simulink model "Lead_Acid_Battery_2021"  (R2024b)
settings: Solver=VariableStepAuto  StartTime=0.0  StopTime=100  RelTol=1e-3
settings Model: Creator=10537  LastModifiedBy=10537

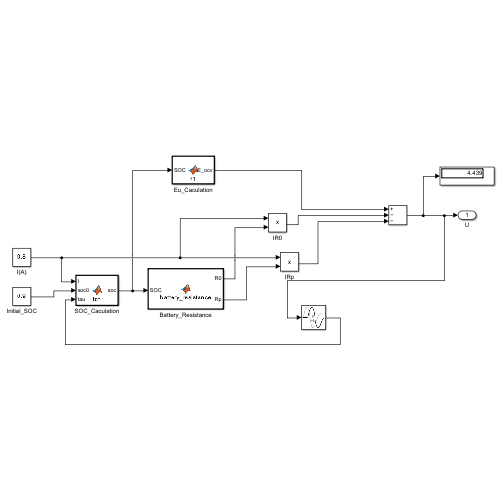
[thumbnail: Simulink's stored preview of the top-level diagram]
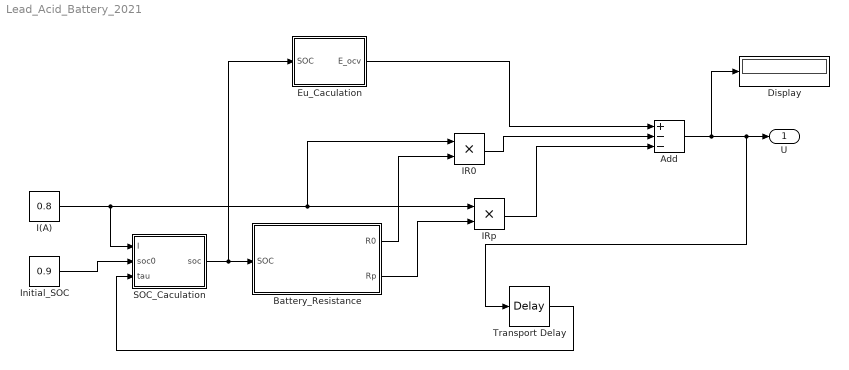
== system Lead_Acid_Battery_2021 ==
  Add : Sum  Inputs=+--
  Battery_Resistance : MATLAB Function  TreatAsAtomicUnit=on
  Display : Display
  Eu_Caculation : MATLAB Function  TreatAsAtomicUnit=on
  I(A) : Constant  Value=0.8
  IR0 : Product
  IRp : Product
  Initial_SOC : Constant  Value=0.9
  SOC_Caculation : MATLAB Function  TreatAsAtomicUnit=on
  Transport Delay : TransportDelay
  U : Outport
  wires:
  Battery_Resistance/1(R0) -> IR0/2
  Battery_Resistance/2(Rp) -> IRp/2
  IR0/1 -> Add/2
  IRp/1 -> Add/3
  Add/1 -> Display/1, Transport Delay/1, U/1
  I(A)/1 -> IRp/1, IR0/1, SOC_Caculation/1(I)
  Initial_SOC/1 -> SOC_Caculation/2(soc0)
  SOC_Caculation/1(soc) -> Eu_Caculation/1(SOC), Battery_Resistance/1(SOC)
  Transport Delay/1 -> SOC_Caculation/3(tau)
  Eu_Caculation/1(E_ocv) -> Add/1

== matlab function Lead_Acid_Battery_2021/Eu_Caculation ==
  data: SOC input; E_ocv output
function E_ocv = f1(SOC)
    % 电池的开路电压E_ocv与SOC的多项式关系
    E_ocv = 3.7 * SOC^3 - 0.8 * SOC^2 + 2.1 * SOC + 1.0;  % 拟合多项式
end

== matlab function Lead_Acid_Battery_2021/Battery_Resistance ==
  data: SOC input; R0 output; Rp output
function [R0, Rp] = battery_resistance(SOC)
    % 电池的欧姆内阻 R0（根据二次曲线拟合）
    a0 = 0.5; a1 = 0.1; a2 = -0.02;  
    R0 = a0 + a1 * SOC + a2 * SOC^2;

    % 电池的极化内阻 Rp（根据指数曲线拟合）
    b0 = 0.05; b1 = 3; b2 = 0.01;  
    Rp = b0 * exp(-b1 * SOC) + b2;
end

== matlab function Lead_Acid_Battery_2021/SOC_Caculation ==
  data: I input; soc output; soc0 input; tau input
function soc = fcn(I, soc0, tau)
    Qn=3.6;
    Ts=1;
    persistent soc_k
    if isempty(soc_k)
        soc_k = soc0;
    end

    % 延迟部分：模拟延迟的SOC
    soc_delayed = soc_k;  % 使用持久的变量 soc_k 作为延迟的SOC
    
    % 根据延迟SOC更新当前的SOC
    soc_k = soc_delayed - I * Ts / (Qn * 3600);
    
    % 限制SOC范围 [0, 1]
    soc_k = min(max(soc_k, 0), 1);
    
    % 返回更新后的SOC
    soc = soc_k;  % 你可以选择将延迟部分的结果作为返回值
end
